simulink model "tone"  (R2016a)
settings: Solver=VariableStepAuto  StartTime=0.0  StopTime=5  RelTol=1e-3
libraries: dspsrcs4 x1
settings Model: Creator=v3best  LastModifiedBy=v3best

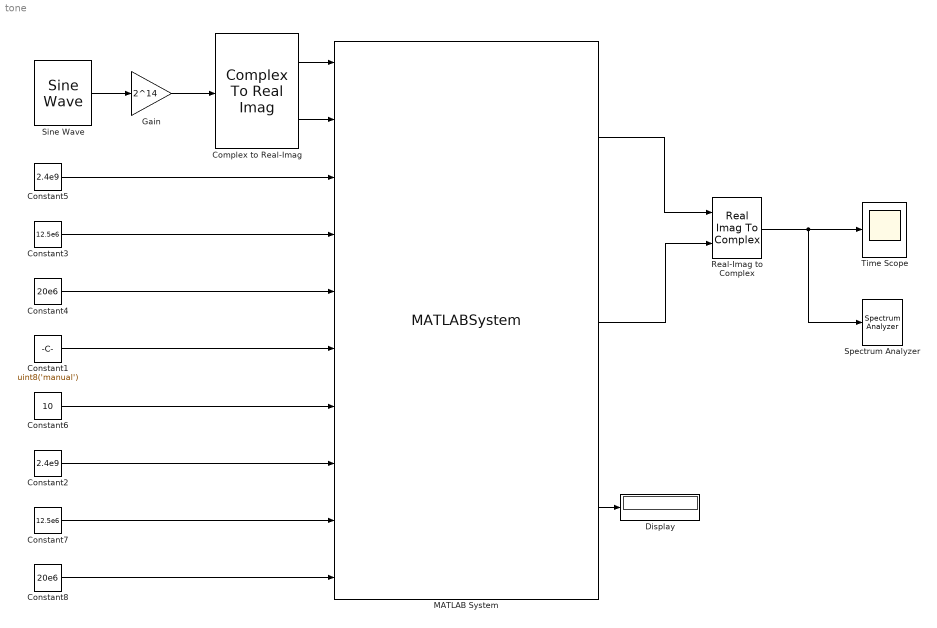
== system tone ==
  Complex to Real-Imag : ComplexToRealImag
  Constant1 : Constant  Value=uint8('manual')  SampleTime=-1
  Constant2 : Constant  Value=2.4e9  SampleTime=-1
  Constant3 : Constant  Value=12.5e6  SampleTime=-1
  Constant4 : Constant  Value=20e6  SampleTime=-1
  Constant5 : Constant  Value=2.4e9  SampleTime=-1
  Constant6 : Constant  Value=10  SampleTime=-1
  Constant7 : Constant  Value=12.5e6  SampleTime=-1
  Constant8 : Constant  Value=20e6  SampleTime=-1
  Display : Display
  Gain : Gain  Gain=2^14
  MATLAB System : MATLABSystem  DialogController=sysobjdialog.BlockDynDialog  System=iio_sys_obj  ip_address=192.168.2.1  dev_name=ad9361  in_ch_no=2  in_ch_size=1e5  out_ch_no=2  out_ch_size=1e5  SimulateUsing=Interpreted execution
      mask Type: iio_sys_obj
      mask Display:
      | disp('ad9361');
      | port_label('input',1,'DATA_IN1');
      | port_label('input',2,'DATA_IN2');
      | port_label('input',3,'RX_LO_FREQ');
      | port_label('input',4,'RX_SAMPLING_FREQ');
      | port_label('input',5,'RX_RF_BANDWIDTH');
      | port_label('input',6,'RX1_GAIN_MODE');
      | port_label('input',7,'RX1_GAIN');
      | port_label('input',8,'TX_LO_FREQ');
      | port_label('input',9,'TX_SAMPLING_FREQ');
      | port_label('input',10,'TX_RF_BANDWIDTH');
      | port_label('output',1,'DATA_OUT1');
      | port_label('output',2,'DATA_OUT2');
      | port_label('output',3,'RX1_RSSI');
  Real-Imag to Complex : RealImagToComplex
  Sine Wave : dspsrcs4/Sine Wave  Amplitude=1  Frequency=100  Phase=0  SampleMode=Discrete  OutComplex=Complex  CompMethod=Trigonometric fcn  TableSize=Speed  SampleTime=1/1e5  SamplesPerFrame=1e4  ResetState=Restart at time zero  OutputFrames=off  dataType=double  wordLen=16  udDataType=sfix(16)  fracBitsMode=Best precision  numFracBits=15  OutDataTypeStr=double  LastOutDataTypeStr=double
  Spectrum Analyzer : SpectrumAnalyzer
  Time Scope : Scope
  wires:
  Sine Wave/1 -> Gain/1
  Complex to Real-Imag/1 -> MATLAB System/1
  Complex to Real-Imag/2 -> MATLAB System/2
  MATLAB System/1 -> Real-Imag to Complex/1
  MATLAB System/2 -> Real-Imag to Complex/2
  Real-Imag to Complex/1 -> Spectrum Analyzer/1, Time Scope/1
  Constant5/1 -> MATLAB System/3
  Constant3/1 -> MATLAB System/4
  Constant4/1 -> MATLAB System/5
  Constant1/1 -> MATLAB System/6
  Constant8/1 -> MATLAB System/10
  Constant2/1 -> MATLAB System/8
  Constant6/1 -> MATLAB System/7
  Constant7/1 -> MATLAB System/9
  Gain/1 -> Complex to Real-Imag/1
  MATLAB System/3 -> Display/1
